simulink model "desired_watcher"  (R2020a)
settings: Solver=VariableStepAuto  StartTime=0.0  StopTime=10.0  RelTol=1e-3
undefined symbols (not defined in the file or in its folder): MAV
libraries: simulink x1
settings Model: Creator=Tamer  LastModifiedBy=Tamer
settings SolverCC: ZeroCrossControl=DisableAll
settings DataIOCC: SaveOutput=off  SaveTime=off
settings GRTTargetCC: CombineOutputUpdateFcns=off  MatFileLogging=off

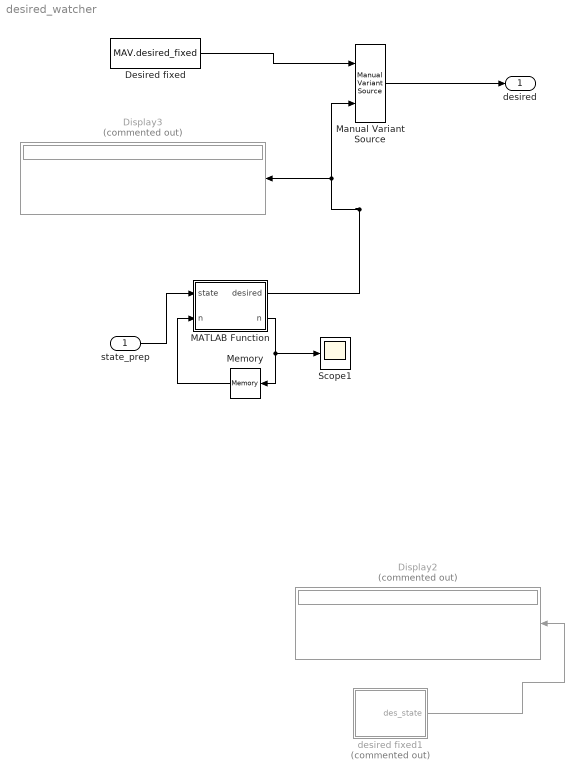
== system desired_watcher ==
  state_prep : Inport  PortDimensions=[15 1]
  Desired fixed : Constant  Value=MAV.desired_fixed
  Display2 : Display  Commented=on
  Display3 : Display  Commented=on
  MATLAB Function : MATLAB Function  TreatAsAtomicUnit=on
  Manual Variant Source : simulink/Signal Routing/Manual Variant Source  NumChoices=2  LabelModeActiveChoice=V_1
  Memory : Memory  InitialCondition=1
  Scope1 : Scope
  desired fixed1 : MATLAB Function  Commented=on  TreatAsAtomicUnit=on
  desired : Outport
  wires:
  MATLAB Function/2(n) -> Scope1/1, Memory/1
  MATLAB Function/1(desired) -> Display3/1, Manual Variant Source/2
  state_prep/1 -> MATLAB Function/1(state)
  Memory/1 -> MATLAB Function/2("n ")
  Desired fixed/1 -> Manual Variant Source/1
  Manual Variant Source/1 -> desired/1
  desired fixed1/1(des_state) -> Display2/1

== matlab function desired_watcher/MATLAB Function ==
  data: state input; desired output; n input; n output
function [desired, n] = fcn(state, n)

x = state(1); y = state(2); z = state(3);
r = [x y z]';

% select r_desired_prev

r_des = get_square_traj(n);
% r_des = get_circle_traj(n);
if norm(r_des - r) < 0.5
    n = n + 1;
%     r_des = get_circle_traj(n);
    r_des = get_square_traj(n);
end

desired = [r_des [3 0 0]' [0 0 0]'];

end

function r_des = get_circle_traj(n)
    R = 10;
    N = 30;
    n = mod(n, N) + 1;
    r_des = [
        R*cos(2*pi/N*n);
        0;
        R*sin(2*pi/N*n) 
    ];
end

function r_des = get_square_traj(n)
    a = 10;
    map = [
        a 0 0; 
        a 0 a;
        0 0 a;
        0 0 0; 
    ]';
    r_des = map(:, mod(n, 4) + 1);
end

== matlab function desired_watcher/desired fixed1 ==
  data: des_state output; MAV parameter
function des_state = fcn(  MAV)

% pos = [8  0 5.87]';
pos = [MAV.x0  MAV.y0 MAV.z0]';
vel = [3 0 0]';
acc = [0 0 0]';
des_state = [pos vel acc];
